simulink model "sym5_6_Level"  (R2021a)
settings: Solver=VariableStepAuto  StartTime=0.0  StopTime=8  RelTol=1e-3
undefined symbols (not defined in the file): lambda2
libraries: dspsigops x13, dspquant2 x1
(part 2 of 4)

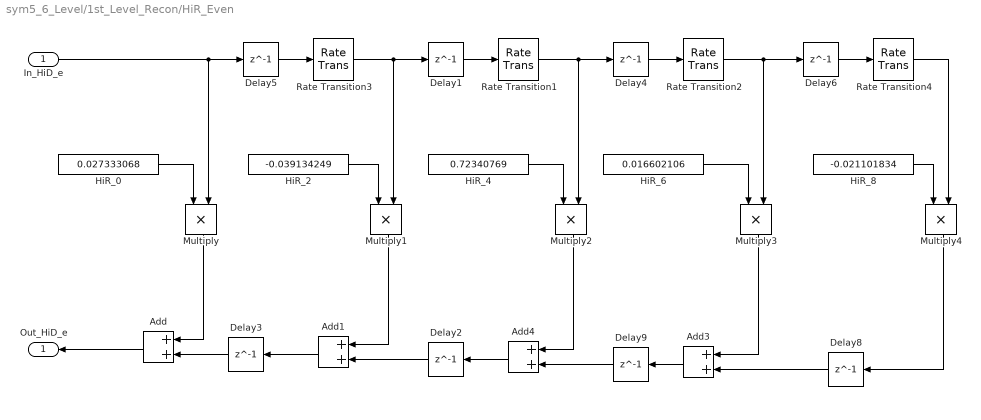
== system sym5_6_Level/1st_Level_Recon/HiR_Even ==
  In_HiD_e : Inport  OutDataTypeStr=double  SampleTime=1/44100
  Add{,1,3..4} (4 alike) : Sum  AccumDataTypeStr=double  OutDataTypeStr=double
  Delay{1..6,8..9} (8 alike) : Delay  DelayLength=1  SampleTime=1/44100
  HiR_0 : Constant  Value=0.027333068  OutDataTypeStr=double  SampleTime=0.000022675736
  HiR_2 : Constant  Value=-0.039134249  OutDataTypeStr=double  SampleTime=0.000022675736
  HiR_4 : Constant  Value=0.72340769  OutDataTypeStr=double  SampleTime=0.000022675736
  HiR_6 : Constant  Value=0.016602106  OutDataTypeStr=double  SampleTime=0.000022675736
  HiR_8 : Constant  Value=-0.021101834  OutDataTypeStr=double  SampleTime=0.000022675736
  Multiply{,1..4} (5 alike) : Product  OutDataTypeStr=double
  Rate Transition{1..4} (4 alike) : RateTransition  OutPortSampleTime=1/44100
  Out_HiD_e : Outport  OutDataTypeStr=double  SampleTime=1/44100  VectorParamsAs1DForOutWhenUnconnected=off
  wires:
  HiR_8/1 -> Multiply4/1
  Add4/1 -> Delay2/1
  Multiply4/1 -> Delay8/1
  HiR_0/1 -> Multiply/1
  Multiply/1 -> Add/1
  Delay3/1 -> Add/2
  Rate Transition2/1 -> Delay6/1, Multiply3/2
  Delay8/1 -> Add3/2
  Delay1/1 -> Rate Transition1/1
  Delay4/1 -> Rate Transition2/1
  Delay6/1 -> Rate Transition4/1
  Rate Transition3/1 -> Delay1/1, Multiply1/2
  Delay5/1 -> Rate Transition3/1
  Delay9/1 -> Add4/2
  Rate Transition4/1 -> Multiply4/2
  Add3/1 -> Delay9/1
  Rate Transition1/1 -> Delay4/1, Multiply2/2
  HiR_6/1 -> Multiply3/1
  HiR_4/1 -> Multiply2/1
  In_HiD_e/1 -> Delay5/1, Multiply/2
  Add1/1 -> Delay3/1
  Add/1 -> Out_HiD_e/1
  Multiply1/1 -> Add1/1
  Multiply3/1 -> Add3/1
  Multiply2/1 -> Add4/1
  Delay2/1 -> Add1/2
  HiR_2/1 -> Multiply1/1

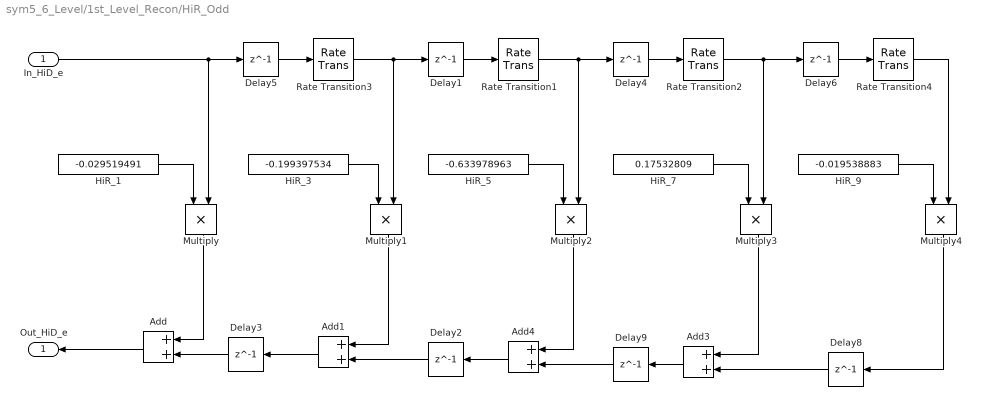
== system sym5_6_Level/1st_Level_Recon/HiR_Odd ==
  In_HiD_e : Inport  OutDataTypeStr=double  SampleTime=1/44100
  Add{,1,3..4} (4 alike) : Sum  AccumDataTypeStr=double  OutDataTypeStr=double
  Delay{1..6,8..9} (8 alike) : Delay  DelayLength=1  SampleTime=1/44100
  HiR_1 : Constant  Value=-0.029519491  OutDataTypeStr=double  SampleTime=0.000022675736
  HiR_3 : Constant  Value=-0.199397534  OutDataTypeStr=double  SampleTime=0.000022675736
  HiR_5 : Constant  Value=-0.633978963  OutDataTypeStr=double  SampleTime=0.000022675736
  HiR_7 : Constant  Value=0.17532809  OutDataTypeStr=double  SampleTime=0.000022675736
  HiR_9 : Constant  Value=-0.019538883  OutDataTypeStr=double  SampleTime=0.000022675736
  Multiply{,1..4} (5 alike) : Product  OutDataTypeStr=double
  Rate Transition{1..4} (4 alike) : RateTransition  OutPortSampleTime=1/44100
  Out_HiD_e : Outport  OutDataTypeStr=double  SampleTime=1/44100  VectorParamsAs1DForOutWhenUnconnected=off
  wires:
  HiR_9/1 -> Multiply4/1
  Add4/1 -> Delay2/1
  Multiply4/1 -> Delay8/1
  HiR_1/1 -> Multiply/1
  Multiply/1 -> Add/1
  Delay3/1 -> Add/2
  Rate Transition2/1 -> Delay6/1, Multiply3/2
  Delay8/1 -> Add3/2
  Delay1/1 -> Rate Transition1/1
  Delay4/1 -> Rate Transition2/1
  Delay6/1 -> Rate Transition4/1
  Rate Transition3/1 -> Delay1/1, Multiply1/2
  Delay5/1 -> Rate Transition3/1
  Delay9/1 -> Add4/2
  Rate Transition4/1 -> Multiply4/2
  Add3/1 -> Delay9/1
  Rate Transition1/1 -> Delay4/1, Multiply2/2
  HiR_7/1 -> Multiply3/1
  HiR_5/1 -> Multiply2/1
  In_HiD_e/1 -> Delay5/1, Multiply/2
  Add1/1 -> Delay3/1
  Add/1 -> Out_HiD_e/1
  Multiply1/1 -> Add1/1
  Multiply3/1 -> Add3/1
  Multiply2/1 -> Add4/1
  Delay2/1 -> Add1/2
  HiR_3/1 -> Multiply1/1

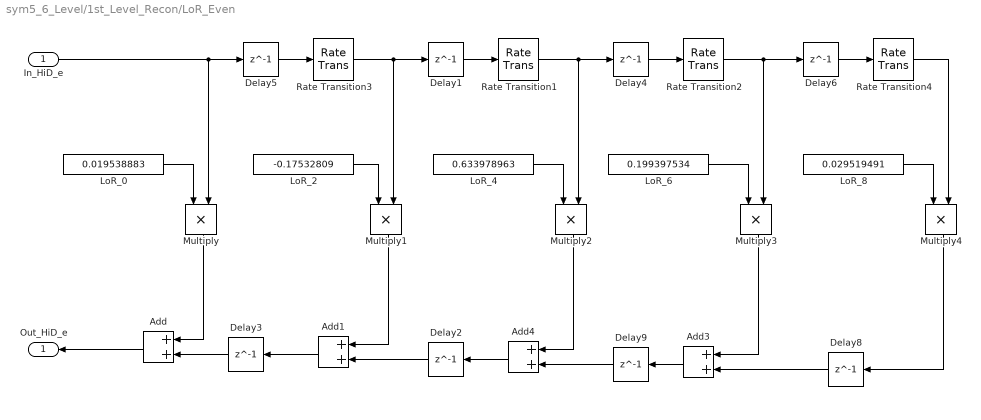
== system sym5_6_Level/1st_Level_Recon/LoR_Even ==
  In_HiD_e : Inport  OutDataTypeStr=double  SampleTime=1/44100
  Add{,1,3..4} (4 alike) : Sum  AccumDataTypeStr=double  OutDataTypeStr=double
  Delay{1..6,8..9} (8 alike) : Delay  DelayLength=1  SampleTime=1/44100
  LoR_0 : Constant  Value=0.019538883  OutDataTypeStr=double  SampleTime=0.000022675736
  LoR_2 : Constant  Value=-0.17532809  OutDataTypeStr=double  SampleTime=0.000022675736
  LoR_4 : Constant  Value=0.633978963  OutDataTypeStr=double  SampleTime=0.000022675736
  LoR_6 : Constant  Value=0.199397534  OutDataTypeStr=double  SampleTime=0.000022675736
  LoR_8 : Constant  Value=0.029519491  OutDataTypeStr=double  SampleTime=0.000022675736
  Multiply{,1..4} (5 alike) : Product  OutDataTypeStr=double
  Rate Transition{1..4} (4 alike) : RateTransition  OutPortSampleTime=1/44100
  Out_HiD_e : Outport  OutDataTypeStr=double  SampleTime=1/44100  VectorParamsAs1DForOutWhenUnconnected=off
  wires:
  LoR_8/1 -> Multiply4/1
  Add4/1 -> Delay2/1
  Multiply4/1 -> Delay8/1
  LoR_0/1 -> Multiply/1
  Multiply/1 -> Add/1
  Delay3/1 -> Add/2
  Rate Transition2/1 -> Delay6/1, Multiply3/2
  Delay8/1 -> Add3/2
  Delay1/1 -> Rate Transition1/1
  Delay4/1 -> Rate Transition2/1
  Delay6/1 -> Rate Transition4/1
  Rate Transition3/1 -> Delay1/1, Multiply1/2
  Delay5/1 -> Rate Transition3/1
  Delay9/1 -> Add4/2
  Rate Transition4/1 -> Multiply4/2
  Add3/1 -> Delay9/1
  Rate Transition1/1 -> Delay4/1, Multiply2/2
  LoR_6/1 -> Multiply3/1
  LoR_4/1 -> Multiply2/1
  In_HiD_e/1 -> Delay5/1, Multiply/2
  Add1/1 -> Delay3/1
  Add/1 -> Out_HiD_e/1
  Multiply1/1 -> Add1/1
  Multiply3/1 -> Add3/1
  Multiply2/1 -> Add4/1
  Delay2/1 -> Add1/2
  LoR_2/1 -> Multiply1/1

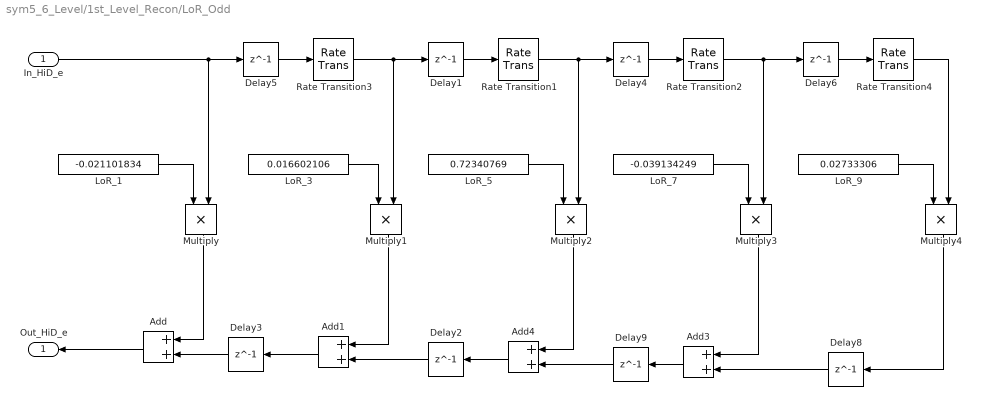
== system sym5_6_Level/1st_Level_Recon/LoR_Odd ==
  In_HiD_e : Inport  OutDataTypeStr=double  SampleTime=1/44100
  Add{,1,3..4} (4 alike) : Sum  AccumDataTypeStr=double  OutDataTypeStr=double
  Delay{1..6,8..9} (8 alike) : Delay  DelayLength=1  SampleTime=1/44100
  LoR_1 : Constant  Value=-0.021101834  OutDataTypeStr=fixdt(1,16,12)  SampleTime=0.000022675736
  LoR_3 : Constant  Value=0.016602106  OutDataTypeStr=fixdt(1,16,12)  SampleTime=0.000022675736
  LoR_5 : Constant  Value=0.72340769  OutDataTypeStr=fixdt(1,16,12)  SampleTime=0.000022675736
  LoR_7 : Constant  Value=-0.039134249  OutDataTypeStr=fixdt(1,16,12)  SampleTime=0.000022675736
  LoR_9 : Constant  Value=0.02733306  OutDataTypeStr=fixdt(1,16,12)  SampleTime=0.000022675736
  Multiply{,1..4} (5 alike) : Product  OutDataTypeStr=double
  Rate Transition{1..4} (4 alike) : RateTransition  OutPortSampleTime=1/44100
  Out_HiD_e : Outport  OutDataTypeStr=double  SampleTime=1/44100  VectorParamsAs1DForOutWhenUnconnected=off
  wires:
  LoR_9/1 -> Multiply4/1
  Add4/1 -> Delay2/1
  Multiply4/1 -> Delay8/1
  LoR_1/1 -> Multiply/1
  Multiply/1 -> Add/1
  Delay3/1 -> Add/2
  Rate Transition2/1 -> Delay6/1, Multiply3/2
  Delay8/1 -> Add3/2
  Delay1/1 -> Rate Transition1/1
  Delay4/1 -> Rate Transition2/1
  Delay6/1 -> Rate Transition4/1
  Rate Transition3/1 -> Delay1/1, Multiply1/2
  Delay5/1 -> Rate Transition3/1
  Delay9/1 -> Add4/2
  Rate Transition4/1 -> Multiply4/2
  Add3/1 -> Delay9/1
  Rate Transition1/1 -> Delay4/1, Multiply2/2
  LoR_7/1 -> Multiply3/1
  LoR_5/1 -> Multiply2/1
  In_HiD_e/1 -> Delay5/1, Multiply/2
  Add1/1 -> Delay3/1
  Add/1 -> Out_HiD_e/1
  Multiply1/1 -> Add1/1
  Multiply3/1 -> Add3/1
  Multiply2/1 -> Add4/1
  Delay2/1 -> Add1/2
  LoR_3/1 -> Multiply1/1

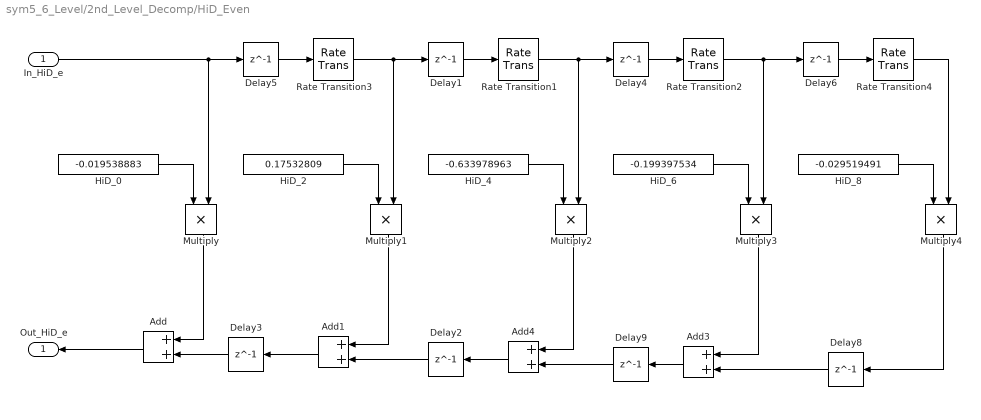
== system sym5_6_Level/2nd_Level_Decomp/HiD_Even ==
  In_HiD_e : Inport  OutDataTypeStr=double  SampleTime=1/44100
  Add{,1,3..4} (4 alike) : Sum  AccumDataTypeStr=double  OutDataTypeStr=double
  Delay{1..6,8..9} (8 alike) : Delay  DelayLength=1  SampleTime=1/44100
  HiD_0 : Constant  Value=-0.019538883  OutDataTypeStr=double  SampleTime=1/44100
  HiD_2 : Constant  Value=0.17532809  OutDataTypeStr=double  SampleTime=1/44100
  HiD_4 : Constant  Value=-0.633978963  OutDataTypeStr=double  SampleTime=1/44100
  HiD_6 : Constant  Value=-0.199397534  OutDataTypeStr=double  SampleTime=1/44100
  HiD_8 : Constant  Value=-0.029519491  OutDataTypeStr=double  SampleTime=1/44100
  Multiply{,1..4} (5 alike) : Product  OutDataTypeStr=double
  Rate Transition{1..4} (4 alike) : RateTransition  OutPortSampleTime=1/44100
  Out_HiD_e : Outport  OutDataTypeStr=double  SampleTime=1/44100  VectorParamsAs1DForOutWhenUnconnected=off
  wires:
  Multiply2/1 -> Add4/1
  Add1/1 -> Delay3/1
  Rate Transition1/1 -> Delay4/1, Multiply2/2
  In_HiD_e/1 -> Delay5/1, Multiply/2
  Delay2/1 -> Add1/2
  Multiply1/1 -> Add1/1
  Rate Transition3/1 -> Delay1/1, Multiply1/2
  Multiply3/1 -> Add3/1
  Add/1 -> Out_HiD_e/1
  Delay3/1 -> Add/2
  Multiply/1 -> Add/1
  HiD_8/1 -> Multiply4/1
  Delay9/1 -> Add4/2
  Rate Transition2/1 -> Delay6/1, Multiply3/2
  Rate Transition4/1 -> Multiply4/2
  Delay8/1 -> Add3/2
  Add3/1 -> Delay9/1
  Add4/1 -> Delay2/1
  HiD_6/1 -> Multiply3/1
  HiD_4/1 -> Multiply2/1
  HiD_2/1 -> Multiply1/1
  HiD_0/1 -> Multiply/1
  Multiply4/1 -> Delay8/1
  Delay6/1 -> Rate Transition4/1
  Delay4/1 -> Rate Transition2/1
  Delay1/1 -> Rate Transition1/1
  Delay5/1 -> Rate Transition3/1

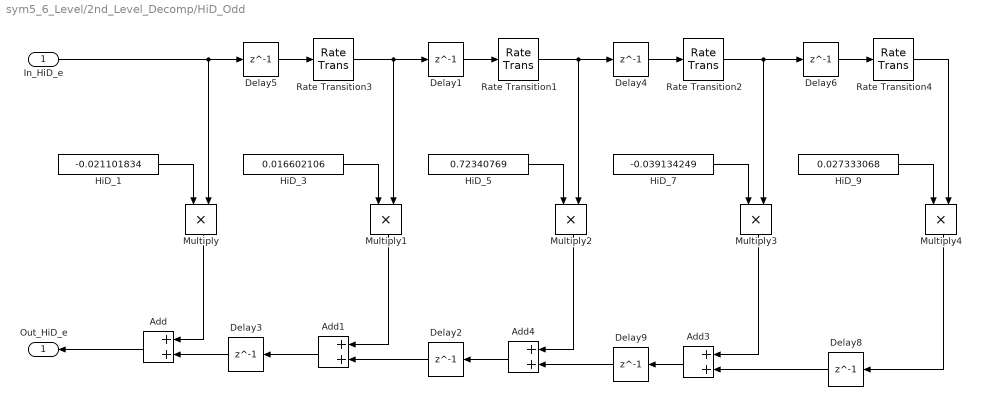
== system sym5_6_Level/2nd_Level_Decomp/HiD_Odd ==
  In_HiD_e : Inport  OutDataTypeStr=double  SampleTime=1/44100
  Add{,1,3..4} (4 alike) : Sum  AccumDataTypeStr=double  OutDataTypeStr=double
  Delay{1..6,8..9} (8 alike) : Delay  DelayLength=1  SampleTime=1/44100
  HiD_1 : Constant  Value=-0.021101834  OutDataTypeStr=double  SampleTime=0.000022675736
  HiD_3 : Constant  Value=0.016602106  OutDataTypeStr=double  SampleTime=0.000022675736
  HiD_5 : Constant  Value=0.72340769  OutDataTypeStr=double  SampleTime=0.000022675736
  HiD_7 : Constant  Value=-0.039134249  OutDataTypeStr=double  SampleTime=0.000022675736
  HiD_9 : Constant  Value=0.027333068  OutDataTypeStr=double  SampleTime=0.000022675736
  Multiply{,1..4} (5 alike) : Product  OutDataTypeStr=double
  Rate Transition{1..4} (4 alike) : RateTransition  OutPortSampleTime=1/44100
  Out_HiD_e : Outport  OutDataTypeStr=double  SampleTime=1/44100  VectorParamsAs1DForOutWhenUnconnected=off
  wires:
  HiD_9/1 -> Multiply4/1
  Add4/1 -> Delay2/1
  Multiply4/1 -> Delay8/1
  HiD_1/1 -> Multiply/1
  Multiply/1 -> Add/1
  Delay3/1 -> Add/2
  Rate Transition2/1 -> Delay6/1, Multiply3/2
  Delay8/1 -> Add3/2
  Delay1/1 -> Rate Transition1/1
  Delay4/1 -> Rate Transition2/1
  Delay6/1 -> Rate Transition4/1
  Rate Transition3/1 -> Delay1/1, Multiply1/2
  Delay5/1 -> Rate Transition3/1
  Delay9/1 -> Add4/2
  Rate Transition4/1 -> Multiply4/2
  Add3/1 -> Delay9/1
  Rate Transition1/1 -> Delay4/1, Multiply2/2
  HiD_7/1 -> Multiply3/1
  HiD_5/1 -> Multiply2/1
  In_HiD_e/1 -> Delay5/1, Multiply/2
  Add1/1 -> Delay3/1
  Add/1 -> Out_HiD_e/1
  Multiply1/1 -> Add1/1
  Multiply3/1 -> Add3/1
  Multiply2/1 -> Add4/1
  Delay2/1 -> Add1/2
  HiD_3/1 -> Multiply1/1

== system sym5_6_Level/2nd_Level_Decomp/LoD_Even ==
  In_HiD_e : Inport  OutDataTypeStr=double  SampleTime=1/44100
  Add{,1,3..4} (4 alike) : Sum  AccumDataTypeStr=double  OutDataTypeStr=double
  Delay{1..6,8..9} (8 alike) : Delay  DelayLength=1  SampleTime=1/44100
  LoD_0 : Constant  Value=0.02733306  OutDataTypeStr=double  SampleTime=0.000022675736
  LoD_2 : Constant  Value=-0.039134249  OutDataTypeStr=double  SampleTime=0.000022675736
  LoD_4 : Constant  Value=0.72340769  OutDataTypeStr=double  SampleTime=0.000022675736
  LoD_6 : Constant  Value=0.016602106  OutDataTypeStr=double  SampleTime=0.000022675736
  LoD_8 : Constant  Value=-0.021101834  OutDataTypeStr=double  SampleTime=0.000022675736
  Multiply{,1..4} (5 alike) : Product  OutDataTypeStr=double
  Rate Transition{1..4} (4 alike) : RateTransition  OutPortSampleTime=1/44100
  Out_HiD_e : Outport  OutDataTypeStr=double  SampleTime=1/44100  VectorParamsAs1DForOutWhenUnconnected=off
  wires:
  LoD_8/1 -> Multiply4/1
  Add4/1 -> Delay2/1
  Multiply4/1 -> Delay8/1
  LoD_0/1 -> Multiply/1
  Multiply/1 -> Add/1
  Delay3/1 -> Add/2
  Rate Transition2/1 -> Delay6/1, Multiply3/2
  Delay8/1 -> Add3/2
  Delay1/1 -> Rate Transition1/1
  Delay4/1 -> Rate Transition2/1
  Delay6/1 -> Rate Transition4/1
  Rate Transition3/1 -> Delay1/1, Multiply1/2
  Delay5/1 -> Rate Transition3/1
  Delay9/1 -> Add4/2
  Rate Transition4/1 -> Multiply4/2
  Add3/1 -> Delay9/1
  Rate Transition1/1 -> Delay4/1, Multiply2/2
  LoD_6/1 -> Multiply3/1
  LoD_4/1 -> Multiply2/1
  In_HiD_e/1 -> Delay5/1, Multiply/2
  Add1/1 -> Delay3/1
  Add/1 -> Out_HiD_e/1
  Multiply1/1 -> Add1/1
  Multiply3/1 -> Add3/1
  Multiply2/1 -> Add4/1
  Delay2/1 -> Add1/2
  LoD_2/1 -> Multiply1/1

== system sym5_6_Level/2nd_Level_Decomp/LoD_Odd ==
  In_HiD_e : Inport  OutDataTypeStr=double  SampleTime=1/44100
  Add{,1,3..4} (4 alike) : Sum  AccumDataTypeStr=double  OutDataTypeStr=double
  Delay{1..6,8..9} (8 alike) : Delay  DelayLength=1  SampleTime=1/44100
  LoD_1 : Constant  Value=0.029519491  OutDataTypeStr=double  SampleTime=0.000022675736
  LoD_3 : Constant  Value=0.199397534  OutDataTypeStr=double  SampleTime=0.000022675736
  LoD_5 : Constant  Value=0.633978963  OutDataTypeStr=double  SampleTime=0.000022675736
  LoD_7 : Constant  Value=-0.17532809  OutDataTypeStr=double  SampleTime=0.000022675736
  LoD_9 : Constant  Value=0.019538883  OutDataTypeStr=double  SampleTime=0.000022675736
  Multiply{,1..4} (5 alike) : Product  OutDataTypeStr=double
  Rate Transition{1..4} (4 alike) : RateTransition  OutPortSampleTime=1/44100
  Out_HiD_e : Outport  OutDataTypeStr=double  SampleTime=1/44100  VectorParamsAs1DForOutWhenUnconnected=off
  wires:
  LoD_9/1 -> Multiply4/1
  Add4/1 -> Delay2/1
  Multiply4/1 -> Delay8/1
  LoD_1/1 -> Multiply/1
  Multiply/1 -> Add/1
  Delay3/1 -> Add/2
  Rate Transition2/1 -> Delay6/1, Multiply3/2
  Delay8/1 -> Add3/2
  Delay1/1 -> Rate Transition1/1
  Delay4/1 -> Rate Transition2/1
  Delay6/1 -> Rate Transition4/1
  Rate Transition3/1 -> Delay1/1, Multiply1/2
  Delay5/1 -> Rate Transition3/1
  Delay9/1 -> Add4/2
  Rate Transition4/1 -> Multiply4/2
  Add3/1 -> Delay9/1
  Rate Transition1/1 -> Delay4/1, Multiply2/2
  LoD_7/1 -> Multiply3/1
  LoD_5/1 -> Multiply2/1
  In_HiD_e/1 -> Delay5/1, Multiply/2
  Add1/1 -> Delay3/1
  Add/1 -> Out_HiD_e/1
  Multiply1/1 -> Add1/1
  Multiply3/1 -> Add3/1
  Multiply2/1 -> Add4/1
  Delay2/1 -> Add1/2
  LoD_3/1 -> Multiply1/1

== system sym5_6_Level/2nd_Level_Recon/HiR_Even ==
  In_HiD_e : Inport  OutDataTypeStr=double  SampleTime=1/44100
  Add{,1,3..4} (4 alike) : Sum  AccumDataTypeStr=double  OutDataTypeStr=double
  Delay{1..6,8..9} (8 alike) : Delay  DelayLength=1  SampleTime=1/44100
  HiR_0 : Constant  Value=0.027333068  OutDataTypeStr=double  SampleTime=0.000022675736
  HiR_2 : Constant  Value=-0.039134249  OutDataTypeStr=double  SampleTime=0.000022675736
  HiR_4 : Constant  Value=0.72340769  OutDataTypeStr=double  SampleTime=0.000022675736
  HiR_6 : Constant  Value=0.016602106  OutDataTypeStr=double  SampleTime=0.000022675736
  HiR_8 : Constant  Value=-0.021101834  OutDataTypeStr=double  SampleTime=0.000022675736
  Multiply{,1..4} (5 alike) : Product  OutDataTypeStr=double
  Rate Transition{1..4} (4 alike) : RateTransition  OutPortSampleTime=1/44100
  Out_HiD_e : Outport  OutDataTypeStr=double  SampleTime=1/44100  VectorParamsAs1DForOutWhenUnconnected=off
  wires:
  HiR_8/1 -> Multiply4/1
  Add4/1 -> Delay2/1
  Multiply4/1 -> Delay8/1
  HiR_0/1 -> Multiply/1
  Multiply/1 -> Add/1
  Delay3/1 -> Add/2
  Rate Transition2/1 -> Delay6/1, Multiply3/2
  Delay8/1 -> Add3/2
  Delay1/1 -> Rate Transition1/1
  Delay4/1 -> Rate Transition2/1
  Delay6/1 -> Rate Transition4/1
  Rate Transition3/1 -> Delay1/1, Multiply1/2
  Delay5/1 -> Rate Transition3/1
  Delay9/1 -> Add4/2
  Rate Transition4/1 -> Multiply4/2
  Add3/1 -> Delay9/1
  Rate Transition1/1 -> Delay4/1, Multiply2/2
  HiR_6/1 -> Multiply3/1
  HiR_4/1 -> Multiply2/1
  In_HiD_e/1 -> Delay5/1, Multiply/2
  Add1/1 -> Delay3/1
  Add/1 -> Out_HiD_e/1
  Multiply1/1 -> Add1/1
  Multiply3/1 -> Add3/1
  Multiply2/1 -> Add4/1
  Delay2/1 -> Add1/2
  HiR_2/1 -> Multiply1/1

== system sym5_6_Level/2nd_Level_Recon/HiR_Odd ==
  In_HiD_e : Inport  OutDataTypeStr=double  SampleTime=1/44100
  Add{,1,3..4} (4 alike) : Sum  AccumDataTypeStr=double  OutDataTypeStr=double
  Delay{1..6,8..9} (8 alike) : Delay  DelayLength=1  SampleTime=1/44100
  HiR_1 : Constant  Value=-0.029519491  OutDataTypeStr=double  SampleTime=0.000022675736
  HiR_3 : Constant  Value=-0.199397534  OutDataTypeStr=double  SampleTime=0.000022675736
  HiR_5 : Constant  Value=-0.633978963  OutDataTypeStr=double  SampleTime=0.000022675736
  HiR_7 : Constant  Value=0.17532809  OutDataTypeStr=double  SampleTime=0.000022675736
  HiR_9 : Constant  Value=-0.019538883  OutDataTypeStr=double  SampleTime=0.000022675736
  Multiply{,1..4} (5 alike) : Product  OutDataTypeStr=double
  Rate Transition{1..4} (4 alike) : RateTransition  OutPortSampleTime=1/44100
  Out_HiD_e : Outport  OutDataTypeStr=double  SampleTime=1/44100  VectorParamsAs1DForOutWhenUnconnected=off
  wires:
  HiR_9/1 -> Multiply4/1
  Add4/1 -> Delay2/1
  Multiply4/1 -> Delay8/1
  HiR_1/1 -> Multiply/1
  Multiply/1 -> Add/1
  Delay3/1 -> Add/2
  Rate Transition2/1 -> Delay6/1, Multiply3/2
  Delay8/1 -> Add3/2
  Delay1/1 -> Rate Transition1/1
  Delay4/1 -> Rate Transition2/1
  Delay6/1 -> Rate Transition4/1
  Rate Transition3/1 -> Delay1/1, Multiply1/2
  Delay5/1 -> Rate Transition3/1
  Delay9/1 -> Add4/2
  Rate Transition4/1 -> Multiply4/2
  Add3/1 -> Delay9/1
  Rate Transition1/1 -> Delay4/1, Multiply2/2
  HiR_7/1 -> Multiply3/1
  HiR_5/1 -> Multiply2/1
  In_HiD_e/1 -> Delay5/1, Multiply/2
  Add1/1 -> Delay3/1
  Add/1 -> Out_HiD_e/1
  Multiply1/1 -> Add1/1
  Multiply3/1 -> Add3/1
  Multiply2/1 -> Add4/1
  Delay2/1 -> Add1/2
  HiR_3/1 -> Multiply1/1

== system sym5_6_Level/2nd_Level_Recon/LoR_Even ==
  In_HiD_e : Inport  OutDataTypeStr=double  SampleTime=1/44100
  Add{,1,3..4} (4 alike) : Sum  AccumDataTypeStr=double  OutDataTypeStr=double
  Delay{1..6,8..9} (8 alike) : Delay  DelayLength=1  SampleTime=1/44100
  LoR_0 : Constant  Value=0.019538883  OutDataTypeStr=double  SampleTime=0.000022675736
  LoR_2 : Constant  Value=-0.17532809  OutDataTypeStr=double  SampleTime=0.000022675736
  LoR_4 : Constant  Value=0.633978963  OutDataTypeStr=double  SampleTime=0.000022675736
  LoR_6 : Constant  Value=0.199397534  OutDataTypeStr=double  SampleTime=0.000022675736
  LoR_8 : Constant  Value=0.029519491  OutDataTypeStr=double  SampleTime=0.000022675736
  Multiply{,1..4} (5 alike) : Product  OutDataTypeStr=double
  Rate Transition{1..4} (4 alike) : RateTransition  OutPortSampleTime=1/44100
  Out_HiD_e : Outport  OutDataTypeStr=double  SampleTime=1/44100  VectorParamsAs1DForOutWhenUnconnected=off
  wires:
  LoR_8/1 -> Multiply4/1
  Add4/1 -> Delay2/1
  Multiply4/1 -> Delay8/1
  LoR_0/1 -> Multiply/1
  Multiply/1 -> Add/1
  Delay3/1 -> Add/2
  Rate Transition2/1 -> Delay6/1, Multiply3/2
  Delay8/1 -> Add3/2
  Delay1/1 -> Rate Transition1/1
  Delay4/1 -> Rate Transition2/1
  Delay6/1 -> Rate Transition4/1
  Rate Transition3/1 -> Delay1/1, Multiply1/2
  Delay5/1 -> Rate Transition3/1
  Delay9/1 -> Add4/2
  Rate Transition4/1 -> Multiply4/2
  Add3/1 -> Delay9/1
  Rate Transition1/1 -> Delay4/1, Multiply2/2
  LoR_6/1 -> Multiply3/1
  LoR_4/1 -> Multiply2/1
  In_HiD_e/1 -> Delay5/1, Multiply/2
  Add1/1 -> Delay3/1
  Add/1 -> Out_HiD_e/1
  Multiply1/1 -> Add1/1
  Multiply3/1 -> Add3/1
  Multiply2/1 -> Add4/1
  Delay2/1 -> Add1/2
  LoR_2/1 -> Multiply1/1

== system sym5_6_Level/2nd_Level_Recon/LoR_Odd ==
  In_HiD_e : Inport  OutDataTypeStr=double  SampleTime=1/44100
  Add{,1,3..4} (4 alike) : Sum  AccumDataTypeStr=double  OutDataTypeStr=double
  Delay{1..6,8..9} (8 alike) : Delay  DelayLength=1  SampleTime=1/44100
  LoR_1 : Constant  Value=-0.021101834  OutDataTypeStr=fixdt(1,16,12)  SampleTime=0.000022675736
  LoR_3 : Constant  Value=0.016602106  OutDataTypeStr=fixdt(1,16,12)  SampleTime=0.000022675736
  LoR_5 : Constant  Value=0.72340769  OutDataTypeStr=fixdt(1,16,12)  SampleTime=0.000022675736
  LoR_7 : Constant  Value=-0.039134249  OutDataTypeStr=fixdt(1,16,12)  SampleTime=0.000022675736
  LoR_9 : Constant  Value=0.02733306  OutDataTypeStr=fixdt(1,16,12)  SampleTime=0.000022675736
  Multiply{,1..4} (5 alike) : Product  OutDataTypeStr=double
  Rate Transition{1..4} (4 alike) : RateTransition  OutPortSampleTime=1/44100
  Out_HiD_e : Outport  OutDataTypeStr=double  SampleTime=1/44100  VectorParamsAs1DForOutWhenUnconnected=off
  wires:
  LoR_9/1 -> Multiply4/1
  Add4/1 -> Delay2/1
  Multiply4/1 -> Delay8/1
  LoR_1/1 -> Multiply/1
  Multiply/1 -> Add/1
  Delay3/1 -> Add/2
  Rate Transition2/1 -> Delay6/1, Multiply3/2
  Delay8/1 -> Add3/2
  Delay1/1 -> Rate Transition1/1
  Delay4/1 -> Rate Transition2/1
  Delay6/1 -> Rate Transition4/1
  Rate Transition3/1 -> Delay1/1, Multiply1/2
  Delay5/1 -> Rate Transition3/1
  Delay9/1 -> Add4/2
  Rate Transition4/1 -> Multiply4/2
  Add3/1 -> Delay9/1
  Rate Transition1/1 -> Delay4/1, Multiply2/2
  LoR_7/1 -> Multiply3/1
  LoR_5/1 -> Multiply2/1
  In_HiD_e/1 -> Delay5/1, Multiply/2
  Add1/1 -> Delay3/1
  Add/1 -> Out_HiD_e/1
  Multiply1/1 -> Add1/1
  Multiply3/1 -> Add3/1
  Multiply2/1 -> Add4/1
  Delay2/1 -> Add1/2
  LoR_3/1 -> Multiply1/1

== system sym5_6_Level/3rd_Level_Decomp/HiD_Even ==
  In_HiD_e : Inport  OutDataTypeStr=double  SampleTime=1/44100
  Add{,1,3..4} (4 alike) : Sum  AccumDataTypeStr=double  OutDataTypeStr=double
  Delay{1..6,8..9} (8 alike) : Delay  DelayLength=1  SampleTime=1/44100
  HiD_0 : Constant  Value=-0.019538883  OutDataTypeStr=double  SampleTime=1/44100
  HiD_2 : Constant  Value=0.17532809  OutDataTypeStr=double  SampleTime=1/44100
  HiD_4 : Constant  Value=-0.633978963  OutDataTypeStr=double  SampleTime=1/44100
  HiD_6 : Constant  Value=-0.199397534  OutDataTypeStr=double  SampleTime=1/44100
  HiD_8 : Constant  Value=-0.029519491  OutDataTypeStr=double  SampleTime=1/44100
  Multiply{,1..4} (5 alike) : Product  OutDataTypeStr=double
  Rate Transition{1..4} (4 alike) : RateTransition  OutPortSampleTime=1/44100
  Out_HiD_e : Outport  OutDataTypeStr=double  SampleTime=1/44100  VectorParamsAs1DForOutWhenUnconnected=off
  wires:
  Multiply2/1 -> Add4/1
  Add1/1 -> Delay3/1
  Rate Transition1/1 -> Delay4/1, Multiply2/2
  In_HiD_e/1 -> Delay5/1, Multiply/2
  Delay2/1 -> Add1/2
  Multiply1/1 -> Add1/1
  Rate Transition3/1 -> Delay1/1, Multiply1/2
  Multiply3/1 -> Add3/1
  Add/1 -> Out_HiD_e/1
  Delay3/1 -> Add/2
  Multiply/1 -> Add/1
  HiD_8/1 -> Multiply4/1
  Delay9/1 -> Add4/2
  Rate Transition2/1 -> Delay6/1, Multiply3/2
  Rate Transition4/1 -> Multiply4/2
  Delay8/1 -> Add3/2
  Add3/1 -> Delay9/1
  Add4/1 -> Delay2/1
  HiD_6/1 -> Multiply3/1
  HiD_4/1 -> Multiply2/1
  HiD_2/1 -> Multiply1/1
  HiD_0/1 -> Multiply/1
  Multiply4/1 -> Delay8/1
  Delay6/1 -> Rate Transition4/1
  Delay4/1 -> Rate Transition2/1
  Delay1/1 -> Rate Transition1/1
  Delay5/1 -> Rate Transition3/1

== system sym5_6_Level/3rd_Level_Decomp/HiD_Odd ==
  In_HiD_e : Inport  OutDataTypeStr=double  SampleTime=1/44100
  Add{,1,3..4} (4 alike) : Sum  AccumDataTypeStr=double  OutDataTypeStr=double
  Delay{1..6,8..9} (8 alike) : Delay  DelayLength=1  SampleTime=1/44100
  HiD_1 : Constant  Value=-0.021101834  OutDataTypeStr=double  SampleTime=0.000022675736
  HiD_3 : Constant  Value=0.016602106  OutDataTypeStr=double  SampleTime=0.000022675736
  HiD_5 : Constant  Value=0.72340769  OutDataTypeStr=double  SampleTime=0.000022675736
  HiD_7 : Constant  Value=-0.039134249  OutDataTypeStr=double  SampleTime=0.000022675736
  HiD_9 : Constant  Value=0.027333068  OutDataTypeStr=double  SampleTime=0.000022675736
  Multiply{,1..4} (5 alike) : Product  OutDataTypeStr=double
  Rate Transition{1..4} (4 alike) : RateTransition  OutPortSampleTime=1/44100
  Out_HiD_e : Outport  OutDataTypeStr=double  SampleTime=1/44100  VectorParamsAs1DForOutWhenUnconnected=off
  wires:
  HiD_9/1 -> Multiply4/1
  Add4/1 -> Delay2/1
  Multiply4/1 -> Delay8/1
  HiD_1/1 -> Multiply/1
  Multiply/1 -> Add/1
  Delay3/1 -> Add/2
  Rate Transition2/1 -> Delay6/1, Multiply3/2
  Delay8/1 -> Add3/2
  Delay1/1 -> Rate Transition1/1
  Delay4/1 -> Rate Transition2/1
  Delay6/1 -> Rate Transition4/1
  Rate Transition3/1 -> Delay1/1, Multiply1/2
  Delay5/1 -> Rate Transition3/1
  Delay9/1 -> Add4/2
  Rate Transition4/1 -> Multiply4/2
  Add3/1 -> Delay9/1
  Rate Transition1/1 -> Delay4/1, Multiply2/2
  HiD_7/1 -> Multiply3/1
  HiD_5/1 -> Multiply2/1
  In_HiD_e/1 -> Delay5/1, Multiply/2
  Add1/1 -> Delay3/1
  Add/1 -> Out_HiD_e/1
  Multiply1/1 -> Add1/1
  Multiply3/1 -> Add3/1
  Multiply2/1 -> Add4/1
  Delay2/1 -> Add1/2
  HiD_3/1 -> Multiply1/1

== system sym5_6_Level/3rd_Level_Decomp/LoD_Even ==
  In_HiD_e : Inport  OutDataTypeStr=double  SampleTime=1/44100
  Add{,1,3..4} (4 alike) : Sum  AccumDataTypeStr=double  OutDataTypeStr=double
  Delay{1..6,8..9} (8 alike) : Delay  DelayLength=1  SampleTime=1/44100
  LoD_0 : Constant  Value=0.02733306  OutDataTypeStr=double  SampleTime=0.000022675736
  LoD_2 : Constant  Value=-0.039134249  OutDataTypeStr=double  SampleTime=0.000022675736
  LoD_4 : Constant  Value=0.72340769  OutDataTypeStr=double  SampleTime=0.000022675736
  LoD_6 : Constant  Value=0.016602106  OutDataTypeStr=double  SampleTime=0.000022675736
  LoD_8 : Constant  Value=-0.021101834  OutDataTypeStr=double  SampleTime=0.000022675736
  Multiply{,1..4} (5 alike) : Product  OutDataTypeStr=double
  Rate Transition{1..4} (4 alike) : RateTransition  OutPortSampleTime=1/44100
  Out_HiD_e : Outport  OutDataTypeStr=double  SampleTime=1/44100  VectorParamsAs1DForOutWhenUnconnected=off
  wires:
  LoD_8/1 -> Multiply4/1
  Add4/1 -> Delay2/1
  Multiply4/1 -> Delay8/1
  LoD_0/1 -> Multiply/1
  Multiply/1 -> Add/1
  Delay3/1 -> Add/2
  Rate Transition2/1 -> Delay6/1, Multiply3/2
  Delay8/1 -> Add3/2
  Delay1/1 -> Rate Transition1/1
  Delay4/1 -> Rate Transition2/1
  Delay6/1 -> Rate Transition4/1
  Rate Transition3/1 -> Delay1/1, Multiply1/2
  Delay5/1 -> Rate Transition3/1
  Delay9/1 -> Add4/2
  Rate Transition4/1 -> Multiply4/2
  Add3/1 -> Delay9/1
  Rate Transition1/1 -> Delay4/1, Multiply2/2
  LoD_6/1 -> Multiply3/1
  LoD_4/1 -> Multiply2/1
  In_HiD_e/1 -> Delay5/1, Multiply/2
  Add1/1 -> Delay3/1
  Add/1 -> Out_HiD_e/1
  Multiply1/1 -> Add1/1
  Multiply3/1 -> Add3/1
  Multiply2/1 -> Add4/1
  Delay2/1 -> Add1/2
  LoD_2/1 -> Multiply1/1

== system sym5_6_Level/3rd_Level_Decomp/LoD_Odd ==
  In_HiD_e : Inport  OutDataTypeStr=double  SampleTime=1/44100
  Add{,1,3..4} (4 alike) : Sum  AccumDataTypeStr=double  OutDataTypeStr=double
  Delay{1..6,8..9} (8 alike) : Delay  DelayLength=1  SampleTime=1/44100
  LoD_1 : Constant  Value=0.029519491  OutDataTypeStr=double  SampleTime=0.000022675736
  LoD_3 : Constant  Value=0.199397534  OutDataTypeStr=double  SampleTime=0.000022675736
  LoD_5 : Constant  Value=0.633978963  OutDataTypeStr=double  SampleTime=0.000022675736
  LoD_7 : Constant  Value=-0.17532809  OutDataTypeStr=double  SampleTime=0.000022675736
  LoD_9 : Constant  Value=0.019538883  OutDataTypeStr=double  SampleTime=0.000022675736
  Multiply{,1..4} (5 alike) : Product  OutDataTypeStr=double
  Rate Transition{1..4} (4 alike) : RateTransition  OutPortSampleTime=1/44100
  Out_HiD_e : Outport  OutDataTypeStr=double  SampleTime=1/44100  VectorParamsAs1DForOutWhenUnconnected=off
  wires:
  LoD_9/1 -> Multiply4/1
  Add4/1 -> Delay2/1
  Multiply4/1 -> Delay8/1
  LoD_1/1 -> Multiply/1
  Multiply/1 -> Add/1
  Delay3/1 -> Add/2
  Rate Transition2/1 -> Delay6/1, Multiply3/2
  Delay8/1 -> Add3/2
  Delay1/1 -> Rate Transition1/1
  Delay4/1 -> Rate Transition2/1
  Delay6/1 -> Rate Transition4/1
  Rate Transition3/1 -> Delay1/1, Multiply1/2
  Delay5/1 -> Rate Transition3/1
  Delay9/1 -> Add4/2
  Rate Transition4/1 -> Multiply4/2
  Add3/1 -> Delay9/1
  Rate Transition1/1 -> Delay4/1, Multiply2/2
  LoD_7/1 -> Multiply3/1
  LoD_5/1 -> Multiply2/1
  In_HiD_e/1 -> Delay5/1, Multiply/2
  Add1/1 -> Delay3/1
  Add/1 -> Out_HiD_e/1
  Multiply1/1 -> Add1/1
  Multiply3/1 -> Add3/1
  Multiply2/1 -> Add4/1
  Delay2/1 -> Add1/2
  LoD_3/1 -> Multiply1/1

== system sym5_6_Level/3rd_Level_Recon/HiR_Even ==
  In_HiD_e : Inport  OutDataTypeStr=double  SampleTime=1/44100
  Add{,1,3..4} (4 alike) : Sum  AccumDataTypeStr=double  OutDataTypeStr=double
  Delay{1..6,8..9} (8 alike) : Delay  DelayLength=1  SampleTime=1/44100
  HiR_0 : Constant  Value=0.027333068  OutDataTypeStr=double  SampleTime=0.000022675736
  HiR_2 : Constant  Value=-0.039134249  OutDataTypeStr=double  SampleTime=0.000022675736
  HiR_4 : Constant  Value=0.72340769  OutDataTypeStr=double  SampleTime=0.000022675736
  HiR_6 : Constant  Value=0.016602106  OutDataTypeStr=double  SampleTime=0.000022675736
  HiR_8 : Constant  Value=-0.021101834  OutDataTypeStr=double  SampleTime=0.000022675736
  Multiply{,1..4} (5 alike) : Product  OutDataTypeStr=double
  Rate Transition{1..4} (4 alike) : RateTransition  OutPortSampleTime=1/44100
  Out_HiD_e : Outport  OutDataTypeStr=double  SampleTime=1/44100  VectorParamsAs1DForOutWhenUnconnected=off
  wires:
  HiR_8/1 -> Multiply4/1
  Add4/1 -> Delay2/1
  Multiply4/1 -> Delay8/1
  HiR_0/1 -> Multiply/1
  Multiply/1 -> Add/1
  Delay3/1 -> Add/2
  Rate Transition2/1 -> Delay6/1, Multiply3/2
  Delay8/1 -> Add3/2
  Delay1/1 -> Rate Transition1/1
  Delay4/1 -> Rate Transition2/1
  Delay6/1 -> Rate Transition4/1
  Rate Transition3/1 -> Delay1/1, Multiply1/2
  Delay5/1 -> Rate Transition3/1
  Delay9/1 -> Add4/2
  Rate Transition4/1 -> Multiply4/2
  Add3/1 -> Delay9/1
  Rate Transition1/1 -> Delay4/1, Multiply2/2
  HiR_6/1 -> Multiply3/1
  HiR_4/1 -> Multiply2/1
  In_HiD_e/1 -> Delay5/1, Multiply/2
  Add1/1 -> Delay3/1
  Add/1 -> Out_HiD_e/1
  Multiply1/1 -> Add1/1
  Multiply3/1 -> Add3/1
  Multiply2/1 -> Add4/1
  Delay2/1 -> Add1/2
  HiR_2/1 -> Multiply1/1

== system sym5_6_Level/3rd_Level_Recon/HiR_Odd ==
  In_HiD_e : Inport  OutDataTypeStr=double  SampleTime=1/44100
  Add{,1,3..4} (4 alike) : Sum  AccumDataTypeStr=double  OutDataTypeStr=double
  Delay{1..6,8..9} (8 alike) : Delay  DelayLength=1  SampleTime=1/44100
  HiR_1 : Constant  Value=-0.029519491  OutDataTypeStr=double  SampleTime=0.000022675736
  HiR_3 : Constant  Value=-0.199397534  OutDataTypeStr=double  SampleTime=0.000022675736
  HiR_5 : Constant  Value=-0.633978963  OutDataTypeStr=double  SampleTime=0.000022675736
  HiR_7 : Constant  Value=0.17532809  OutDataTypeStr=double  SampleTime=0.000022675736
  HiR_9 : Constant  Value=-0.019538883  OutDataTypeStr=double  SampleTime=0.000022675736
  Multiply{,1..4} (5 alike) : Product  OutDataTypeStr=double
  Rate Transition{1..4} (4 alike) : RateTransition  OutPortSampleTime=1/44100
  Out_HiD_e : Outport  OutDataTypeStr=double  SampleTime=1/44100  VectorParamsAs1DForOutWhenUnconnected=off
  wires:
  HiR_9/1 -> Multiply4/1
  Add4/1 -> Delay2/1
  Multiply4/1 -> Delay8/1
  HiR_1/1 -> Multiply/1
  Multiply/1 -> Add/1
  Delay3/1 -> Add/2
  Rate Transition2/1 -> Delay6/1, Multiply3/2
  Delay8/1 -> Add3/2
  Delay1/1 -> Rate Transition1/1
  Delay4/1 -> Rate Transition2/1
  Delay6/1 -> Rate Transition4/1
  Rate Transition3/1 -> Delay1/1, Multiply1/2
  Delay5/1 -> Rate Transition3/1
  Delay9/1 -> Add4/2
  Rate Transition4/1 -> Multiply4/2
  Add3/1 -> Delay9/1
  Rate Transition1/1 -> Delay4/1, Multiply2/2
  HiR_7/1 -> Multiply3/1
  HiR_5/1 -> Multiply2/1
  In_HiD_e/1 -> Delay5/1, Multiply/2
  Add1/1 -> Delay3/1
  Add/1 -> Out_HiD_e/1
  Multiply1/1 -> Add1/1
  Multiply3/1 -> Add3/1
  Multiply2/1 -> Add4/1
  Delay2/1 -> Add1/2
  HiR_3/1 -> Multiply1/1

== system sym5_6_Level/3rd_Level_Recon/LoR_Even ==
  In_HiD_e : Inport  OutDataTypeStr=double  SampleTime=1/44100
  Add{,1,3..4} (4 alike) : Sum  AccumDataTypeStr=double  OutDataTypeStr=double
  Delay{1..6,8..9} (8 alike) : Delay  DelayLength=1  SampleTime=1/44100
  LoR_0 : Constant  Value=0.019538883  OutDataTypeStr=double  SampleTime=0.000022675736
  LoR_2 : Constant  Value=-0.17532809  OutDataTypeStr=double  SampleTime=0.000022675736
  LoR_4 : Constant  Value=0.633978963  OutDataTypeStr=double  SampleTime=0.000022675736
  LoR_6 : Constant  Value=0.199397534  OutDataTypeStr=double  SampleTime=0.000022675736
  LoR_8 : Constant  Value=0.029519491  OutDataTypeStr=double  SampleTime=0.000022675736
  Multiply{,1..4} (5 alike) : Product  OutDataTypeStr=double
  Rate Transition{1..4} (4 alike) : RateTransition  OutPortSampleTime=1/44100
  Out_HiD_e : Outport  OutDataTypeStr=double  SampleTime=1/44100  VectorParamsAs1DForOutWhenUnconnected=off
  wires:
  LoR_8/1 -> Multiply4/1
  Add4/1 -> Delay2/1
  Multiply4/1 -> Delay8/1
  LoR_0/1 -> Multiply/1
  Multiply/1 -> Add/1
  Delay3/1 -> Add/2
  Rate Transition2/1 -> Delay6/1, Multiply3/2
  Delay8/1 -> Add3/2
  Delay1/1 -> Rate Transition1/1
  Delay4/1 -> Rate Transition2/1
  Delay6/1 -> Rate Transition4/1
  Rate Transition3/1 -> Delay1/1, Multiply1/2
  Delay5/1 -> Rate Transition3/1
  Delay9/1 -> Add4/2
  Rate Transition4/1 -> Multiply4/2
  Add3/1 -> Delay9/1
  Rate Transition1/1 -> Delay4/1, Multiply2/2
  LoR_6/1 -> Multiply3/1
  LoR_4/1 -> Multiply2/1
  In_HiD_e/1 -> Delay5/1, Multiply/2
  Add1/1 -> Delay3/1
  Add/1 -> Out_HiD_e/1
  Multiply1/1 -> Add1/1
  Multiply3/1 -> Add3/1
  Multiply2/1 -> Add4/1
  Delay2/1 -> Add1/2
  LoR_2/1 -> Multiply1/1

== system sym5_6_Level/3rd_Level_Recon/LoR_Odd ==
  In_HiD_e : Inport  OutDataTypeStr=double  SampleTime=1/44100
  Add{,1,3..4} (4 alike) : Sum  AccumDataTypeStr=double  OutDataTypeStr=double
  Delay{1..6,8..9} (8 alike) : Delay  DelayLength=1  SampleTime=1/44100
  LoR_1 : Constant  Value=-0.021101834  OutDataTypeStr=fixdt(1,16,12)  SampleTime=0.000022675736
  LoR_3 : Constant  Value=0.016602106  OutDataTypeStr=fixdt(1,16,12)  SampleTime=0.000022675736
  LoR_5 : Constant  Value=0.72340769  OutDataTypeStr=fixdt(1,16,12)  SampleTime=0.000022675736
  LoR_7 : Constant  Value=-0.039134249  OutDataTypeStr=fixdt(1,16,12)  SampleTime=0.000022675736
  LoR_9 : Constant  Value=0.02733306  OutDataTypeStr=fixdt(1,16,12)  SampleTime=0.000022675736
  Multiply{,1..4} (5 alike) : Product  OutDataTypeStr=double
  Rate Transition{1..4} (4 alike) : RateTransition  OutPortSampleTime=1/44100
  Out_HiD_e : Outport  OutDataTypeStr=double  SampleTime=1/44100  VectorParamsAs1DForOutWhenUnconnected=off
  wires:
  LoR_9/1 -> Multiply4/1
  Add4/1 -> Delay2/1
  Multiply4/1 -> Delay8/1
  LoR_1/1 -> Multiply/1
  Multiply/1 -> Add/1
  Delay3/1 -> Add/2
  Rate Transition2/1 -> Delay6/1, Multiply3/2
  Delay8/1 -> Add3/2
  Delay1/1 -> Rate Transition1/1
  Delay4/1 -> Rate Transition2/1
  Delay6/1 -> Rate Transition4/1
  Rate Transition3/1 -> Delay1/1, Multiply1/2
  Delay5/1 -> Rate Transition3/1
  Delay9/1 -> Add4/2
  Rate Transition4/1 -> Multiply4/2
  Add3/1 -> Delay9/1
  Rate Transition1/1 -> Delay4/1, Multiply2/2
  LoR_7/1 -> Multiply3/1
  LoR_5/1 -> Multiply2/1
  In_HiD_e/1 -> Delay5/1, Multiply/2
  Add1/1 -> Delay3/1
  Add/1 -> Out_HiD_e/1
  Multiply1/1 -> Add1/1
  Multiply3/1 -> Add3/1
  Multiply2/1 -> Add4/1
  Delay2/1 -> Add1/2
  LoR_3/1 -> Multiply1/1

== system sym5_6_Level/4th_Level_Decomp/HiD_Even ==
  In_HiD_e : Inport  OutDataTypeStr=double  SampleTime=1/44100
  Add{,1,3..4} (4 alike) : Sum  AccumDataTypeStr=double  OutDataTypeStr=double
  Delay{1..6,8..9} (8 alike) : Delay  DelayLength=1  SampleTime=1/44100
  HiD_0 : Constant  Value=-0.019538883  OutDataTypeStr=double  SampleTime=1/44100
  HiD_2 : Constant  Value=0.17532809  OutDataTypeStr=double  SampleTime=1/44100
  HiD_4 : Constant  Value=-0.633978963  OutDataTypeStr=double  SampleTime=1/44100
  HiD_6 : Constant  Value=-0.199397534  OutDataTypeStr=double  SampleTime=1/44100
  HiD_8 : Constant  Value=-0.029519491  OutDataTypeStr=double  SampleTime=1/44100
  Multiply{,1..4} (5 alike) : Product  OutDataTypeStr=double
  Rate Transition{1..4} (4 alike) : RateTransition  OutPortSampleTime=1/44100
  Out_HiD_e : Outport  OutDataTypeStr=double  SampleTime=1/44100  VectorParamsAs1DForOutWhenUnconnected=off
  wires:
  Multiply2/1 -> Add4/1
  Add1/1 -> Delay3/1
  Rate Transition1/1 -> Delay4/1, Multiply2/2
  In_HiD_e/1 -> Delay5/1, Multiply/2
  Delay2/1 -> Add1/2
  Multiply1/1 -> Add1/1
  Rate Transition3/1 -> Delay1/1, Multiply1/2
  Multiply3/1 -> Add3/1
  Add/1 -> Out_HiD_e/1
  Delay3/1 -> Add/2
  Multiply/1 -> Add/1
  HiD_8/1 -> Multiply4/1
  Delay9/1 -> Add4/2
  Rate Transition2/1 -> Delay6/1, Multiply3/2
  Rate Transition4/1 -> Multiply4/2
  Delay8/1 -> Add3/2
  Add3/1 -> Delay9/1
  Add4/1 -> Delay2/1
  HiD_6/1 -> Multiply3/1
  HiD_4/1 -> Multiply2/1
  HiD_2/1 -> Multiply1/1
  HiD_0/1 -> Multiply/1
  Multiply4/1 -> Delay8/1
  Delay6/1 -> Rate Transition4/1
  Delay4/1 -> Rate Transition2/1
  Delay1/1 -> Rate Transition1/1
  Delay5/1 -> Rate Transition3/1

== system sym5_6_Level/4th_Level_Decomp/HiD_Odd ==
  In_HiD_e : Inport  OutDataTypeStr=double  SampleTime=1/44100
  Add{,1,3..4} (4 alike) : Sum  AccumDataTypeStr=double  OutDataTypeStr=double
  Delay{1..6,8..9} (8 alike) : Delay  DelayLength=1  SampleTime=1/44100
  HiD_1 : Constant  Value=-0.021101834  OutDataTypeStr=double  SampleTime=0.000022675736
  HiD_3 : Constant  Value=0.016602106  OutDataTypeStr=double  SampleTime=0.000022675736
  HiD_5 : Constant  Value=0.72340769  OutDataTypeStr=double  SampleTime=0.000022675736
  HiD_7 : Constant  Value=-0.039134249  OutDataTypeStr=double  SampleTime=0.000022675736
  HiD_9 : Constant  Value=0.027333068  OutDataTypeStr=double  SampleTime=0.000022675736
  Multiply{,1..4} (5 alike) : Product  OutDataTypeStr=double
  Rate Transition{1..4} (4 alike) : RateTransition  OutPortSampleTime=1/44100
  Out_HiD_e : Outport  OutDataTypeStr=double  SampleTime=1/44100  VectorParamsAs1DForOutWhenUnconnected=off
  wires:
  HiD_9/1 -> Multiply4/1
  Add4/1 -> Delay2/1
  Multiply4/1 -> Delay8/1
  HiD_1/1 -> Multiply/1
  Multiply/1 -> Add/1
  Delay3/1 -> Add/2
  Rate Transition2/1 -> Delay6/1, Multiply3/2
  Delay8/1 -> Add3/2
  Delay1/1 -> Rate Transition1/1
  Delay4/1 -> Rate Transition2/1
  Delay6/1 -> Rate Transition4/1
  Rate Transition3/1 -> Delay1/1, Multiply1/2
  Delay5/1 -> Rate Transition3/1
  Delay9/1 -> Add4/2
  Rate Transition4/1 -> Multiply4/2
  Add3/1 -> Delay9/1
  Rate Transition1/1 -> Delay4/1, Multiply2/2
  HiD_7/1 -> Multiply3/1
  HiD_5/1 -> Multiply2/1
  In_HiD_e/1 -> Delay5/1, Multiply/2
  Add1/1 -> Delay3/1
  Add/1 -> Out_HiD_e/1
  Multiply1/1 -> Add1/1
  Multiply3/1 -> Add3/1
  Multiply2/1 -> Add4/1
  Delay2/1 -> Add1/2
  HiD_3/1 -> Multiply1/1

== system sym5_6_Level/4th_Level_Decomp/LoD_Even ==
  In_HiD_e : Inport  OutDataTypeStr=double  SampleTime=1/44100
  Add{,1,3..4} (4 alike) : Sum  AccumDataTypeStr=double  OutDataTypeStr=double
  Delay{1..6,8..9} (8 alike) : Delay  DelayLength=1  SampleTime=1/44100
  LoD_0 : Constant  Value=0.02733306  OutDataTypeStr=double  SampleTime=0.000022675736
  LoD_2 : Constant  Value=-0.039134249  OutDataTypeStr=double  SampleTime=0.000022675736
  LoD_4 : Constant  Value=0.72340769  OutDataTypeStr=double  SampleTime=0.000022675736
  LoD_6 : Constant  Value=0.016602106  OutDataTypeStr=double  SampleTime=0.000022675736
  LoD_8 : Constant  Value=-0.021101834  OutDataTypeStr=double  SampleTime=0.000022675736
  Multiply{,1..4} (5 alike) : Product  OutDataTypeStr=double
  Rate Transition{1..4} (4 alike) : RateTransition  OutPortSampleTime=1/44100
  Out_HiD_e : Outport  OutDataTypeStr=double  SampleTime=1/44100  VectorParamsAs1DForOutWhenUnconnected=off
  wires:
  LoD_8/1 -> Multiply4/1
  Add4/1 -> Delay2/1
  Multiply4/1 -> Delay8/1
  LoD_0/1 -> Multiply/1
  Multiply/1 -> Add/1
  Delay3/1 -> Add/2
  Rate Transition2/1 -> Delay6/1, Multiply3/2
  Delay8/1 -> Add3/2
  Delay1/1 -> Rate Transition1/1
  Delay4/1 -> Rate Transition2/1
  Delay6/1 -> Rate Transition4/1
  Rate Transition3/1 -> Delay1/1, Multiply1/2
  Delay5/1 -> Rate Transition3/1
  Delay9/1 -> Add4/2
  Rate Transition4/1 -> Multiply4/2
  Add3/1 -> Delay9/1
  Rate Transition1/1 -> Delay4/1, Multiply2/2
  LoD_6/1 -> Multiply3/1
  LoD_4/1 -> Multiply2/1
  In_HiD_e/1 -> Delay5/1, Multiply/2
  Add1/1 -> Delay3/1
  Add/1 -> Out_HiD_e/1
  Multiply1/1 -> Add1/1
  Multiply3/1 -> Add3/1
  Multiply2/1 -> Add4/1
  Delay2/1 -> Add1/2
  LoD_2/1 -> Multiply1/1

== system sym5_6_Level/4th_Level_Decomp/LoD_Odd ==
  In_HiD_e : Inport  OutDataTypeStr=double  SampleTime=1/44100
  Add{,1,3..4} (4 alike) : Sum  AccumDataTypeStr=double  OutDataTypeStr=double
  Delay{1..6,8..9} (8 alike) : Delay  DelayLength=1  SampleTime=1/44100
  LoD_1 : Constant  Value=0.029519491  OutDataTypeStr=double  SampleTime=0.000022675736
  LoD_3 : Constant  Value=0.199397534  OutDataTypeStr=double  SampleTime=0.000022675736
  LoD_5 : Constant  Value=0.633978963  OutDataTypeStr=double  SampleTime=0.000022675736
  LoD_7 : Constant  Value=-0.17532809  OutDataTypeStr=double  SampleTime=0.000022675736
  LoD_9 : Constant  Value=0.019538883  OutDataTypeStr=double  SampleTime=0.000022675736
  Multiply{,1..4} (5 alike) : Product  OutDataTypeStr=double
  Rate Transition{1..4} (4 alike) : RateTransition  OutPortSampleTime=1/44100
  Out_HiD_e : Outport  OutDataTypeStr=double  SampleTime=1/44100  VectorParamsAs1DForOutWhenUnconnected=off
  wires:
  LoD_9/1 -> Multiply4/1
  Add4/1 -> Delay2/1
  Multiply4/1 -> Delay8/1
  LoD_1/1 -> Multiply/1
  Multiply/1 -> Add/1
  Delay3/1 -> Add/2
  Rate Transition2/1 -> Delay6/1, Multiply3/2
  Delay8/1 -> Add3/2
  Delay1/1 -> Rate Transition1/1
  Delay4/1 -> Rate Transition2/1
  Delay6/1 -> Rate Transition4/1
  Rate Transition3/1 -> Delay1/1, Multiply1/2
  Delay5/1 -> Rate Transition3/1
  Delay9/1 -> Add4/2
  Rate Transition4/1 -> Multiply4/2
  Add3/1 -> Delay9/1
  Rate Transition1/1 -> Delay4/1, Multiply2/2
  LoD_7/1 -> Multiply3/1
  LoD_5/1 -> Multiply2/1
  In_HiD_e/1 -> Delay5/1, Multiply/2
  Add1/1 -> Delay3/1
  Add/1 -> Out_HiD_e/1
  Multiply1/1 -> Add1/1
  Multiply3/1 -> Add3/1
  Multiply2/1 -> Add4/1
  Delay2/1 -> Add1/2
  LoD_3/1 -> Multiply1/1

== system sym5_6_Level/4th_Level_Recon/HiR_Even ==
  In_HiD_e : Inport  OutDataTypeStr=double  SampleTime=1/44100
  Add{,1,3..4} (4 alike) : Sum  AccumDataTypeStr=double  OutDataTypeStr=double
  Delay{1..6,8..9} (8 alike) : Delay  DelayLength=1  SampleTime=1/44100
  HiR_0 : Constant  Value=0.027333068  OutDataTypeStr=double  SampleTime=0.000022675736
  HiR_2 : Constant  Value=-0.039134249  OutDataTypeStr=double  SampleTime=0.000022675736
  HiR_4 : Constant  Value=0.72340769  OutDataTypeStr=double  SampleTime=0.000022675736
  HiR_6 : Constant  Value=0.016602106  OutDataTypeStr=double  SampleTime=0.000022675736
  HiR_8 : Constant  Value=-0.021101834  OutDataTypeStr=double  SampleTime=0.000022675736
  Multiply{,1..4} (5 alike) : Product  OutDataTypeStr=double
  Rate Transition{1..4} (4 alike) : RateTransition  OutPortSampleTime=1/44100
  Out_HiD_e : Outport  OutDataTypeStr=double  SampleTime=1/44100  VectorParamsAs1DForOutWhenUnconnected=off
  wires:
  HiR_8/1 -> Multiply4/1
  Add4/1 -> Delay2/1
  Multiply4/1 -> Delay8/1
  HiR_0/1 -> Multiply/1
  Multiply/1 -> Add/1
  Delay3/1 -> Add/2
  Rate Transition2/1 -> Delay6/1, Multiply3/2
  Delay8/1 -> Add3/2
  Delay1/1 -> Rate Transition1/1
  Delay4/1 -> Rate Transition2/1
  Delay6/1 -> Rate Transition4/1
  Rate Transition3/1 -> Delay1/1, Multiply1/2
  Delay5/1 -> Rate Transition3/1
  Delay9/1 -> Add4/2
  Rate Transition4/1 -> Multiply4/2
  Add3/1 -> Delay9/1
  Rate Transition1/1 -> Delay4/1, Multiply2/2
  HiR_6/1 -> Multiply3/1
  HiR_4/1 -> Multiply2/1
  In_HiD_e/1 -> Delay5/1, Multiply/2
  Add1/1 -> Delay3/1
  Add/1 -> Out_HiD_e/1
  Multiply1/1 -> Add1/1
  Multiply3/1 -> Add3/1
  Multiply2/1 -> Add4/1
  Delay2/1 -> Add1/2
  HiR_2/1 -> Multiply1/1

== system sym5_6_Level/4th_Level_Recon/HiR_Odd ==
  In_HiD_e : Inport  OutDataTypeStr=double  SampleTime=1/44100
  Add{,1,3..4} (4 alike) : Sum  AccumDataTypeStr=double  OutDataTypeStr=double
  Delay{1..6,8..9} (8 alike) : Delay  DelayLength=1  SampleTime=1/44100
  HiR_1 : Constant  Value=-0.029519491  OutDataTypeStr=double  SampleTime=0.000022675736
  HiR_3 : Constant  Value=-0.199397534  OutDataTypeStr=double  SampleTime=0.000022675736
  HiR_5 : Constant  Value=-0.633978963  OutDataTypeStr=double  SampleTime=0.000022675736
  HiR_7 : Constant  Value=0.17532809  OutDataTypeStr=double  SampleTime=0.000022675736
  HiR_9 : Constant  Value=-0.019538883  OutDataTypeStr=double  SampleTime=0.000022675736
  Multiply{,1..4} (5 alike) : Product  OutDataTypeStr=double
  Rate Transition{1..4} (4 alike) : RateTransition  OutPortSampleTime=1/44100
  Out_HiD_e : Outport  OutDataTypeStr=double  SampleTime=1/44100  VectorParamsAs1DForOutWhenUnconnected=off
  wires:
  HiR_9/1 -> Multiply4/1
  Add4/1 -> Delay2/1
  Multiply4/1 -> Delay8/1
  HiR_1/1 -> Multiply/1
  Multiply/1 -> Add/1
  Delay3/1 -> Add/2
  Rate Transition2/1 -> Delay6/1, Multiply3/2
  Delay8/1 -> Add3/2
  Delay1/1 -> Rate Transition1/1
  Delay4/1 -> Rate Transition2/1
  Delay6/1 -> Rate Transition4/1
  Rate Transition3/1 -> Delay1/1, Multiply1/2
  Delay5/1 -> Rate Transition3/1
  Delay9/1 -> Add4/2
  Rate Transition4/1 -> Multiply4/2
  Add3/1 -> Delay9/1
  Rate Transition1/1 -> Delay4/1, Multiply2/2
  HiR_7/1 -> Multiply3/1
  HiR_5/1 -> Multiply2/1
  In_HiD_e/1 -> Delay5/1, Multiply/2
  Add1/1 -> Delay3/1
  Add/1 -> Out_HiD_e/1
  Multiply1/1 -> Add1/1
  Multiply3/1 -> Add3/1
  Multiply2/1 -> Add4/1
  Delay2/1 -> Add1/2
  HiR_3/1 -> Multiply1/1

== system sym5_6_Level/4th_Level_Recon/LoR_Even ==
  In_HiD_e : Inport  OutDataTypeStr=double  SampleTime=1/44100
  Add{,1,3..4} (4 alike) : Sum  AccumDataTypeStr=double  OutDataTypeStr=double
  Delay{1..6,8..9} (8 alike) : Delay  DelayLength=1  SampleTime=1/44100
  LoR_0 : Constant  Value=0.019538883  OutDataTypeStr=double  SampleTime=0.000022675736
  LoR_2 : Constant  Value=-0.17532809  OutDataTypeStr=double  SampleTime=0.000022675736
  LoR_4 : Constant  Value=0.633978963  OutDataTypeStr=double  SampleTime=0.000022675736
  LoR_6 : Constant  Value=0.199397534  OutDataTypeStr=double  SampleTime=0.000022675736
  LoR_8 : Constant  Value=0.029519491  OutDataTypeStr=double  SampleTime=0.000022675736
  Multiply{,1..4} (5 alike) : Product  OutDataTypeStr=double
  Rate Transition{1..4} (4 alike) : RateTransition  OutPortSampleTime=1/44100
  Out_HiD_e : Outport  OutDataTypeStr=double  SampleTime=1/44100  VectorParamsAs1DForOutWhenUnconnected=off
  wires:
  LoR_8/1 -> Multiply4/1
  Add4/1 -> Delay2/1
  Multiply4/1 -> Delay8/1
  LoR_0/1 -> Multiply/1
  Multiply/1 -> Add/1
  Delay3/1 -> Add/2
  Rate Transition2/1 -> Delay6/1, Multiply3/2
  Delay8/1 -> Add3/2
  Delay1/1 -> Rate Transition1/1
  Delay4/1 -> Rate Transition2/1
  Delay6/1 -> Rate Transition4/1
  Rate Transition3/1 -> Delay1/1, Multiply1/2
  Delay5/1 -> Rate Transition3/1
  Delay9/1 -> Add4/2
  Rate Transition4/1 -> Multiply4/2
  Add3/1 -> Delay9/1
  Rate Transition1/1 -> Delay4/1, Multiply2/2
  LoR_6/1 -> Multiply3/1
  LoR_4/1 -> Multiply2/1
  In_HiD_e/1 -> Delay5/1, Multiply/2
  Add1/1 -> Delay3/1
  Add/1 -> Out_HiD_e/1
  Multiply1/1 -> Add1/1
  Multiply3/1 -> Add3/1
  Multiply2/1 -> Add4/1
  Delay2/1 -> Add1/2
  LoR_2/1 -> Multiply1/1

== system sym5_6_Level/4th_Level_Recon/LoR_Odd ==
  In_HiD_e : Inport  OutDataTypeStr=double  SampleTime=1/44100
  Add{,1,3..4} (4 alike) : Sum  AccumDataTypeStr=double  OutDataTypeStr=double
  Delay{1..6,8..9} (8 alike) : Delay  DelayLength=1  SampleTime=1/44100
  LoR_1 : Constant  Value=-0.021101834  OutDataTypeStr=fixdt(1,16,12)  SampleTime=0.000022675736
  LoR_3 : Constant  Value=0.016602106  OutDataTypeStr=fixdt(1,16,12)  SampleTime=0.000022675736
  LoR_5 : Constant  Value=0.72340769  OutDataTypeStr=fixdt(1,16,12)  SampleTime=0.000022675736
  LoR_7 : Constant  Value=-0.039134249  OutDataTypeStr=fixdt(1,16,12)  SampleTime=0.000022675736
  LoR_9 : Constant  Value=0.02733306  OutDataTypeStr=fixdt(1,16,12)  SampleTime=0.000022675736
  Multiply{,1..4} (5 alike) : Product  OutDataTypeStr=double
  Rate Transition{1..4} (4 alike) : RateTransition  OutPortSampleTime=1/44100
  Out_HiD_e : Outport  OutDataTypeStr=double  SampleTime=1/44100  VectorParamsAs1DForOutWhenUnconnected=off
  wires:
  LoR_9/1 -> Multiply4/1
  Add4/1 -> Delay2/1
  Multiply4/1 -> Delay8/1
  LoR_1/1 -> Multiply/1
  Multiply/1 -> Add/1
  Delay3/1 -> Add/2
  Rate Transition2/1 -> Delay6/1, Multiply3/2
  Delay8/1 -> Add3/2
  Delay1/1 -> Rate Transition1/1
  Delay4/1 -> Rate Transition2/1
  Delay6/1 -> Rate Transition4/1
  Rate Transition3/1 -> Delay1/1, Multiply1/2
  Delay5/1 -> Rate Transition3/1
  Delay9/1 -> Add4/2
  Rate Transition4/1 -> Multiply4/2
  Add3/1 -> Delay9/1
  Rate Transition1/1 -> Delay4/1, Multiply2/2
  LoR_7/1 -> Multiply3/1
  LoR_5/1 -> Multiply2/1
  In_HiD_e/1 -> Delay5/1, Multiply/2
  Add1/1 -> Delay3/1
  Add/1 -> Out_HiD_e/1
  Multiply1/1 -> Add1/1
  Multiply3/1 -> Add3/1
  Multiply2/1 -> Add4/1
  Delay2/1 -> Add1/2
  LoR_3/1 -> Multiply1/1
